simulink model "test_svn"  (R2020b)
settings: Solver=VariableStepAuto  StartTime=0.0  StopTime=10.0  RelTol=1e-3
model workspace (MAT data in the model file):
  a = 0
  b = 1
settings Model: Creator=WYD-PC  LastModifiedBy=WYD-PC

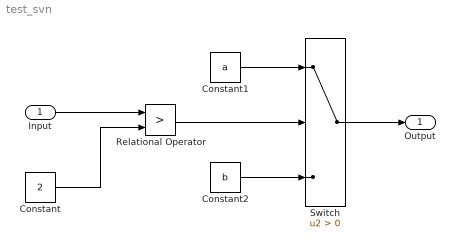
== system test_svn ==
  Input : Inport
  Constant : Constant  Value=2
  Constant1 : Constant  Value=a
  Constant2 : Constant  Value=b
  Relational Operator : RelationalOperator  Operator=>  OutDataTypeStr=boolean  RndMeth=Simplest
  Switch : Switch  Criteria=u2 > Threshold
  Output : Outport
  wires:
  Input/1 -> Relational Operator/1
  Constant/1 -> Relational Operator/2
  Relational Operator/1 -> Switch/2
  Constant1/1 -> Switch/1
  Constant2/1 -> Switch/3
  Switch/1 -> Output/1
